simulink model "Reservoir2Turbine2"  (R2024a)
settings: Solver=ode45  StartTime=0.0  StopTime=200  FixedStep=dt  RelTol=1e-3
undefined symbols (not defined in the file): Cv, D, Dir, Dm, Dp, Ds, eta, f, g, H, Hg, Hir, Hp, Hr, Ht, Hw, Kvsgd, Kvsgp, Lir, Lp, nominal_power, Pa, Pdist_initial, Pg_star_inital, Pgen_inital, Pload_initial, rho, Sn, uv_initial, v, wgen_nom, wgridref, x0
settings Model: PacingRate=100  Creator=tommy  LastModifiedBy=23277
settings RTWCC: GPUComputeCapability=3.5

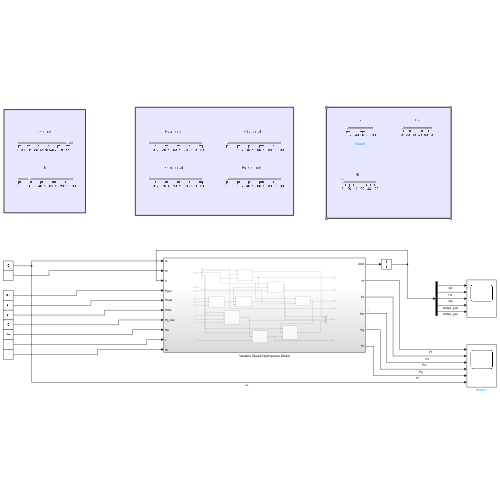
[thumbnail: Simulink's stored preview of the top-level diagram]
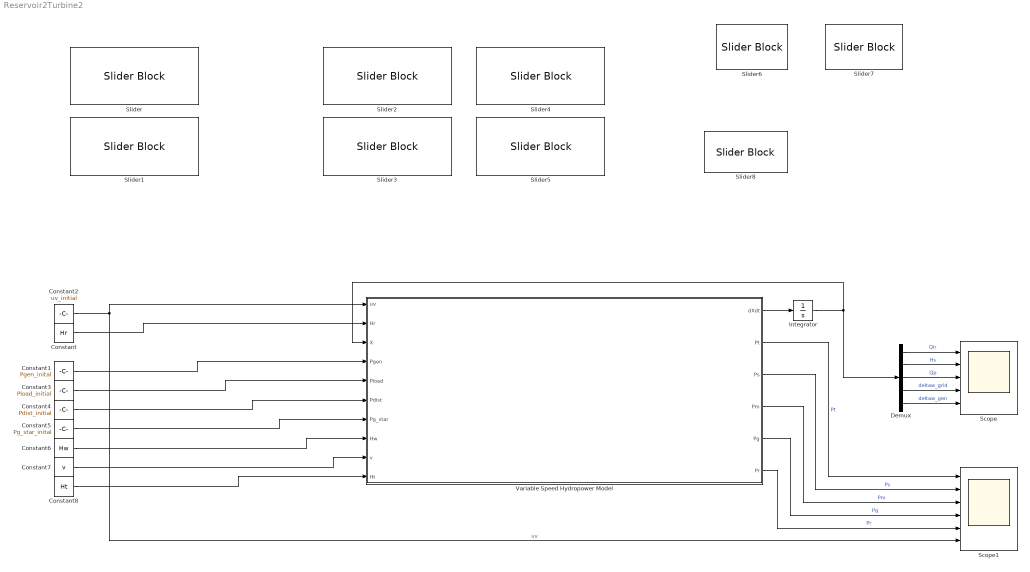
== system Reservoir2Turbine2 ==
  Constant : Constant  Value=Hr
  Constant1 : Constant  Value=Pgen_inital
  Constant2 : Constant  Value=uv_initial
  Constant3 : Constant  Value=Pload_initial
  Constant4 : Constant  Value=Pdist_initial
  Constant5 : Constant  Value=Pg_star_inital
  Constant6 : Constant  Value=Hw
  Constant7 : Constant  Value=v
  Constant8 : Constant  Value=Ht
  Demux : Demux  Outputs=5
  Integrator : Integrator  InitialCondition=x0
  Scope : Scope  NumInputPorts=5
  Scope1 : Scope  NumInputPorts=6
  Slider : SliderBlock  ScaleMax=1
  Slider{1..8} (8 alike) : SliderBlock
  Variable Speed Hydropower Model : Subsystem
  wires:
  Constant2/1 -> Scope1/6, Variable Speed Hydropower Model/1(uv)  "uv"
  Constant/1 -> Variable Speed Hydropower Model/2(Hr)
  Variable Speed Hydropower Model/1(dXdt) -> Integrator/1
  Integrator/1 -> Demux/1, Variable Speed Hydropower Model/3(X)
  Constant1/1 -> Variable Speed Hydropower Model/4(Pgen)
  Constant3/1 -> Variable Speed Hydropower Model/5(Pload)
  Constant4/1 -> Variable Speed Hydropower Model/6(Pdist)
  Constant5/1 -> Variable Speed Hydropower Model/7(Pg_star)
  Demux/1 -> Scope/1  "Qir"
  Demux/2 -> Scope/2  "Hs"
  Demux/3 -> Scope/3  "Qp"
  Demux/4 -> Scope/4  "deltaw_grid"
  Demux/5 -> Scope/5  "deltaw_gen"
  Variable Speed Hydropower Model/2(Pt) -> Scope1/1  "Pt"
  Variable Speed Hydropower Model/3(Ps) -> Scope1/2  "Ps"
  Variable Speed Hydropower Model/4(Pm) -> Scope1/3  "Pm"
  Variable Speed Hydropower Model/5(Pg) -> Scope1/4  "Pg"
  Variable Speed Hydropower Model/6(Pr) -> Scope1/5  "Pr"
  Constant6/1 -> Variable Speed Hydropower Model/8(Hw)
  Constant7/1 -> Variable Speed Hydropower Model/9(v)
  Constant8/1 -> Variable Speed Hydropower Model/10(Ht)

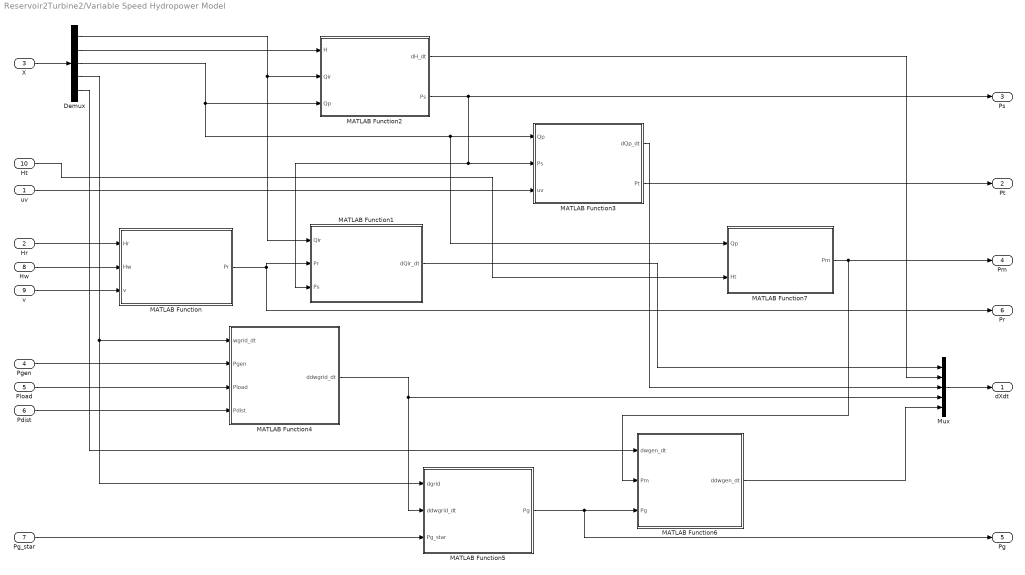
== system Reservoir2Turbine2/Variable Speed Hydropower Model ==
  uv : Inport
  Hr : Inport  Port=2
  X : Inport  Port=3
  Pgen : Inport  Port=4
  Pload : Inport  Port=5
  Pdist : Inport  Port=6
  Pg_star : Inport  Port=7
  Hw : Inport  Port=8
  v : Inport  Port=9
  Ht : Inport  Port=10
  Demux : Demux  Outputs=5
  MATLAB Function : MATLAB Function  TreatAsAtomicUnit=on
  MATLAB Function1 : MATLAB Function  TreatAsAtomicUnit=on
  MATLAB Function2 : MATLAB Function  TreatAsAtomicUnit=on
  MATLAB Function3 : MATLAB Function  TreatAsAtomicUnit=on
  MATLAB Function4 : MATLAB Function  TreatAsAtomicUnit=on
  MATLAB Function5 : MATLAB Function  TreatAsAtomicUnit=on
  MATLAB Function6 : MATLAB Function  TreatAsAtomicUnit=on
  MATLAB Function7 : MATLAB Function  TreatAsAtomicUnit=on
  Mux : Mux  Inputs=5
  dXdt : Outport
  Pt : Outport  Port=2
  Ps : Outport  Port=3
  Pm : Outport  Port=4
  Pg : Outport  Port=5
  Pr : Outport  Port=6
  wires:
  MATLAB Function2/1(dH_dt) -> Mux/2
  MATLAB Function/1(Pr) -> MATLAB Function1/2(Pr), Pr/1
  Mux/1 -> dXdt/1
  Hr/1 -> MATLAB Function/1(Hr)
  MATLAB Function1/1(dQir_dt) -> Mux/1
  MATLAB Function3/1(dQp_dt) -> Mux/3
  uv/1 -> MATLAB Function3/3(uv)
  Demux/1 -> MATLAB Function1/1(Qir), MATLAB Function2/2(Qir)
  Demux/2 -> MATLAB Function2/1(H)
  X/1 -> Demux/1
  MATLAB Function2/2(Ps) -> Ps/1, MATLAB Function3/2(Ps), MATLAB Function1/3(Ps)
  Pgen/1 -> MATLAB Function4/2(Pgen)
  Pload/1 -> MATLAB Function4/3(Pload)
  Pdist/1 -> MATLAB Function4/4(Pdist)
  MATLAB Function4/1(ddwgrid_dt) -> MATLAB Function5/2(ddwgrid_dt), Mux/4
  Demux/3 -> MATLAB Function2/3(Qp), MATLAB Function3/1(Qp), MATLAB Function7/1(Qp)
  Demux/4 -> MATLAB Function5/1(dgrid), MATLAB Function4/1(wgrid_dt)
  Pg_star/1 -> MATLAB Function5/3(Pg_star)
  MATLAB Function5/1(Pg) -> Pg/1, MATLAB Function6/3(Pg)
  MATLAB Function3/2(Pt) -> Pt/1
  MATLAB Function7/1(Pm) -> Pm/1, MATLAB Function6/2(Pm)
  Demux/5 -> MATLAB Function6/1(dwgen_dt)
  MATLAB Function6/1(ddwgen_dt) -> Mux/5
  Hw/1 -> MATLAB Function/2(Hw)
  v/1 -> MATLAB Function/3(v)
  Ht/1 -> MATLAB Function7/2(Ht)

== matlab function Reservoir2Turbine2/Variable Speed Hydropower Model/MATLAB Function6 ==
  data: dwgen_dt input; ddwgen_dt output; Pm input; Pg input; D parameter; wgen_nom parameter; nominal_power parameter; H parameter
function ddwgen_dt = fcn(dwgen_dt, Pm, Pg, D, wgen_nom, nominal_power, H)

pm_pu = Pm/nominal_power;
wgen = dwgen_dt + wgen_nom; % wgen_nom should be wgrid according to equation!

ddwgen_dt = 1/(2*H*wgen)*(pm_pu - Pg - D * dwgen_dt);

== matlab function Reservoir2Turbine2/Variable Speed Hydropower Model/MATLAB Function7 ==
  data: Qp input; Pm output; Ht input; eta parameter; rho parameter; g parameter
function Pm = turbine_model(Qp, Ht, eta, rho, g)

Pm = rho*g*Qp*Ht*eta;                   % Mechanical powe

== matlab function Reservoir2Turbine2/Variable Speed Hydropower Model/MATLAB Function1 ==
  data: Qir input; Pr input; dQir_dt output; Ps input; rho parameter; g parameter; f parameter; Hir parameter; Lir parameter; Dir parameter
function dQir_dt = inlet_race_model(Qir, Pr, Ps, rho, g, f, Hir, Lir, Dir)

    % Geometry
    Air = pi*(Dir/2)^2;          % Area of cross section of inlet pipe

    % Inlet race differential equation (volumetric flow)
    dQir_dt = Air/(rho*Lir)*(Pr - Ps) - pi*Dir*f/(8*Air^2)*Qir*abs(Qir) + g*Air*Hir/Lir;

== matlab function Reservoir2Turbine2/Variable Speed Hydropower Model/MATLAB Function ==
  data: Hr input; Pr output; rho parameter; g parameter; Hw input; v input
function Pr = reservoir_model(Hr, rho, g, Hw, v)

Pr = rho*g*(Hr-v^2/(2*g)-Hw);                % Pressure start of inlet race

== matlab function Reservoir2Turbine2/Variable Speed Hydropower Model/MATLAB Function2 ==
  data: H input; Qir input; dH_dt output; Qp input; Ds parameter; Ps output; Pa parameter; rho parameter; g parameter
function [dH_dt, Ps] = surge_tank_model(H, Qir, Qp, Ds, Pa, rho, g)

    % Geometry
    As = pi*(Ds/2)^2;            % Area of cross section of surge tank

    % Algebraic equations
    Qs = (Qir - Qp);             % Volumetric flow into surge tank
    Ps = Pa + rho*g*H;           % Pressure at end of inlet race

    % Surge tank differential equation (surge tank water height)
    dH_dt = Qs/As;

== matlab function Reservoir2Turbine2/Variable Speed Hydropower Model/MATLAB Function3 ==
  data: Qp input; Ps input; dQp_dt output; uv input; rho parameter; g parameter; f parameter; Cv parameter; Hp parameter; Lp parameter; Dp parameter; Pa parameter; Pt output
function [dQp_dt, Pt] = penstock_model(Qp, Ps, uv, rho, g, f, Cv, Hp, Lp, Dp, Pa)

    % Geometry
    Ap = pi*(Dp/2)^2;            % Area of cross section of penstock pipe

    % Algebraic equations
    Pt = Pa*(1 + (Qp/(Cv*uv))^2);    % Pressure at end of penstock

    % Penstock differential equation (volumetric  flow)
    dQp_dt = Ap/(rho*Lp)*(Ps - Pt) - pi*Dp*f/(8*Ap^2)*Qp*abs(Qp) + g*Ap*Hp/Lp;

== matlab function Reservoir2Turbine2/Variable Speed Hydropower Model/MATLAB Function4 ==
  data: wgrid_dt input; Pgen input; ddwgrid_dt output; Pload input; Pdist input; wgridref parameter; Hg parameter; Sn parameter; Dm parameter
function ddwgrid_dt = grid_model(wgrid_dt, Pgen, Pload, Pdist, wgridref, Hg, Sn, Dm)


ddwgrid_dt = wgridref/(2*Hg*Sn)*(Pgen - Pload + Pdist - Dm*wgrid_dt);

== matlab function Reservoir2Turbine2/Variable Speed Hydropower Model/MATLAB Function5 ==
  data: dgrid input; Pg output; ddwgrid_dt input; Pg_star input; Kvsgp parameter; Kvsgd parameter
function Pg = vsg_model(dgrid, ddwgrid_dt, Pg_star, Kvsgp, Kvsgd)

Pg = Kvsgp*dgrid + Kvsgd*ddwgrid_dt + Pg_star;
